simulink library "EmotorLib"  (R2024b)
settings: Solver=VariableStepAuto  StartTime=0.0  StopTime=10.0  RelTol=1e-3
undefined symbols (not defined in the file or in its folder): electricDrive
libraries: fl_lib x56, nesl_utility x11, ee_lib x2
settings Model: Creator=jjha  LastModifiedBy=jjha
settings OptimizationCC: ReuseModelBlockBuffer=off
settings RTWCC: GPUComputeCapability=3.5

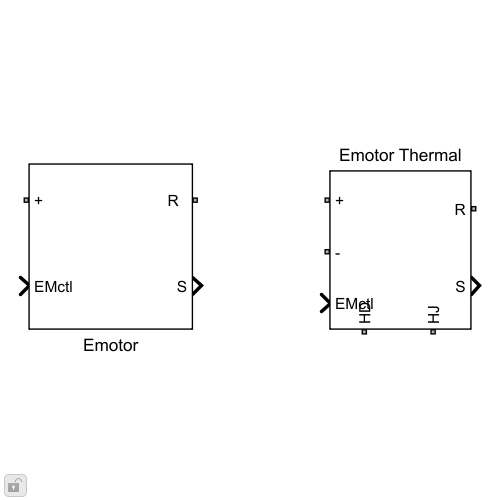
[thumbnail: Simulink's stored preview of the top-level diagram]
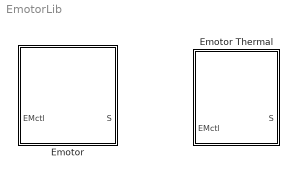
== system EmotorLib ==
  Emotor : Subsystem  mask{max_torque=220, max_power=50000, Tctc=0.002, spMat=[500,10000], tqMat=[10,200], lossMat=[0 0;0 0]}
      mask prompts: max_torque "Max Torque"; max_power "Max Powe"; Tctc "Torque Control Time Constant"; spMat "Speed Vector (rpm)"; tqMat "TorqueVector (Nm)"; lossMat "Losses (W)"
      settings: PortSchema="{\"entries\":[{\"content\":{\"sides\":[{\"content\":{\"connectorIds\":[\"LConn1\",\"In1\"]},\"type\":\"ConnectorPlacement.EquallySpacedRectSide\",\"uuid\":\"4c01f4e7-db0d-4a8e-9bf8-0007797f2983\"},{\"content\":{\"connectorIds\":[\"RConn1\",\"Out1\"],\"side\":\"RIGHT\"},\"type\":\"ConnectorPlacement.EquallySpacedRectSide\",\"uuid\":\"016ff73d-d921-4c23-b0f0-ceb092773eb0\"},{\"content\":{\"connectorIds\":[],\"side\":\"TOP\"},\"type\":\"ConnectorPlacement.EquallySpacedRectSide\",\"uuid\":\"4629c7d5-cdf8-4573-9adc-69c84e237e94\"}]},\"type\":\"ConnectorPlacement.EquallySpacedConnector\",\"uuid\":\"4efbbf6b-ce98-44e7-ad85-9bcf934dac12\"}],\"packageUris\":[\"http://schema.mathworks.com/mf0/Connector/R2020b\"],\"version\":\"1.0\"}"
      mask DialogControl ElecTorque Prompt: Electrical Torque Parameters
      mask DialogControl ElecLosses Prompt: Electrical Losses Parameter
  Emotor Thermal : Subsystem  mask{InitTemp=298.15, IronSpHeat=447, CopperSpHeat=385, IronThConductivity=50, GrossToothMass=0.4836, WindingMass=0.4464, max_torque=220, max_power=50000, Tctc=0.002, spMat=[500,10000], tqMat=[10,200], lossMat=[0 0;0 0], StatorBackIronMass=1.997, StatorRootDia=0.1521, stator_od=0.19812, StatorWindingOhArea=0.0538, Bridgemass=0.0698, rotor_od=.12997, rotorStackLength=0.1516, RotorBackIronMass=16.3802, RotorAreaER=0.0265, RotorAreaCyl=0.0619}
      mask prompts: InitTemp "Initial Temperature(K)"; IronSpHeat "Specific Heat Iron(J/(K*kg))"; CopperSpHeat "Specific Heat Copper(J/(K*kg))"; IronThConductivity "Thermal Conductivity Iron(W/(K*m))"; GrossToothMass "Stator Teeth Mass(kg)"; WindingMass "Stator Winding Mass(kg)"; max_torque "Max Torque"; max_power "Max Power"; Tctc "Torque Control Time Constant"; spMat "Speed Vector (rpm)"; tqMat "TorqueVector (Nm)"; lossMat "Losses (W)"; StatorBackIronMass "Stator Back Iron Mass(kg)"; StatorRootDia "Stator Inner Diameter (m)"; stator_od "Stator Outer Diameter(m)"; StatorWindingOhArea "Stator Winding Area(m^2)"; Bridgemass "Magnet Mass(kg)"; rotor_od "Rotor Outer Diameter(m)"; rotorStackLength "Stack Length(m)"; RotorBackIronMass "Rotor Iron Mass(kg)"; RotorAreaER "Rotor Area ER(m^2)"; RotorAreaCyl "Rotor Cylinder Area(m^2)"
      settings: PortSchema="{\"entries\":[{\"content\":{\"sides\":[{\"content\":{\"connectorIds\":[\"LConn1\",\"LConn2\",\"In1\"]},\"type\":\"ConnectorPlacement.EquallySpacedRectSide\",\"uuid\":\"10df522d-563d-4b08-8533-b994fdc6485c\"},{\"content\":{\"connectorIds\":[\"RConn1\",\"Out1\"],\"side\":\"RIGHT\"},\"type\":\"ConnectorPlacement.EquallySpacedRectSide\",\"uuid\":\"49c7f672-865f-471b-9e0c-89a8670e12b9\"},{\"content\":{\"connectorIds\":[],\"side\":\"TOP\"},\"type\":\"ConnectorPlacement.EquallySpacedRectSide\",\"uuid\":\"483d1bb0-f2a2-4e3e-b03d-59043e33c561\"},{\"content\":{\"connectorIds\":[\"RConn2\",\"RConn3\"],\"side\":\"BOTTOM\"},\"type\":\"ConnectorPlacement.EquallySpacedRectSide\",\"uuid\":\"9824884f-8ef8-4acd-9b94-f9f251c18df1\"}]},\"type\":\"ConnectorPlacement.EquallySpacedConnector\",\"uuid\":\"fbb57d51-9a3c-403f-b1bb-2fd61ef310af\"}],\"packageUris\":[\"http://schema.mathworks.com/mf0/Connector/R2020b\"],\"version\":\"1.0\"}"
      mask DialogControl Container5 Prompt: Electrical Parameters
      mask DialogControl ElecTorque Prompt: Electrical Torque Parameters
      mask DialogControl ElecLosses Prompt: Electrical Losses Parameter
      mask DialogControl Container6 Prompt: Thermal Parameters
      mask DialogControl Container8 Prompt: Rotor
      mask DialogControl Container7 Prompt: Stator

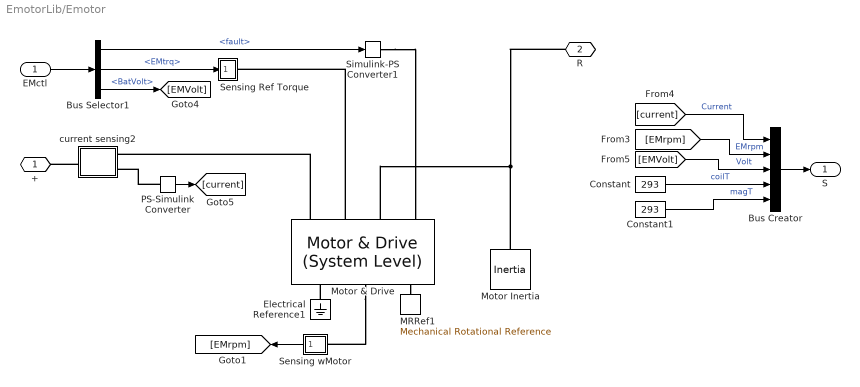
== system EmotorLib/Emotor ==
  EMctl : Inport
  Bus Creator : BusCreator  Inputs=5
  Bus Selector1 : BusSelector  OutputSignals=fault,EMtrq,BatVolt
  Constant : Constant  Value=293
  Constant1 : Constant  Value=293
  Electrical Reference1 : fl_lib/Electrical/Electrical Elements/Electrical Reference
  MRRef1 : fl_lib/Mechanical/Rotational Elements/Mechanical Rotational Reference
  Motor & Drive : ee_lib/Electromechanical/Motor & Drive (System Level)  torque_speed_param=2  overtorque_param=ee.enum.electromech.overtorque.no  T_t=[max_torque max_torque max_torque 0] N*m  T_t_intermittent=[.36, .32, .28, 0] N*m  T_t_2D=[.09, .09, .09; .08, .08, .08; .07, .07, .07; 0, 0, 0] N*m  T_t_intermittent_2D=[.36, .36, .36; .32, .32, .32; .28, .28, .28; 0, 0, 0] N*m  w_t=[ 0 3.75e+3 7.5e+3 8e+3 ] rpm  vdc_t=[6, 12, 24] V  torque_max=max_torque N*m  power_max=max_power W  torque_max_intermittent=0.4 N*m  power_max_intermittent=120 W  time_overtorque=30 s  time_recover=60 s  Tc=Tctc s  EnableSwitch=simscape.enum.onoff.on  losses_param=2  eff=96  w_eff=1500 rpm  T_eff=50 N*m  Piron=200 W  Pbase=0 W  w_eff_vec=spMat rpm  T_eff_vec=tqMat N*m  v_eff_vec=[100, 250, 400] V  losses_mat=lossMat W  efficiency_mat=[95 95 95 95; 95 95 95 95; 95 95 95 95; 95 95 95 95; 95 95 95 95]  losses_mat_3D=ones(5, 4, 3) W  efficiency_mat_3D=95 * ones(5, 4, 3)  Res=0 Ohm  J=0 kg*m^2  lam=1e-5 N*m/(rad/s)  speed0=0 rpm  fault_condition=1  fault_threshold=0.5  faulted_specify=off  faulted_priority=None  faulted=0  faulted_nominal_specify=off  faulted_nominal_value=1  faulted_nominal_unit=1  isSwitchedOff_specify=off  isSwitchedOff_priority=None  isSwitchedOff=0  isSwitchedOff_nominal_specify=off  isSwitchedOff_nominal_value=1  isSwitchedOff_nominal_unit=1  torqueLimitContinuous_specify=off  torqueLimitContinuous_priority=None  torqueLimitContinuous=0 N*m  torqueLimitContinuous_nominal_specify=off  torqueLimitContinuous_nominal_value=1  torqueLimitContinuous_nominal_unit=N*m  alpha=3.93e-3 1/K  Tmeas=25 degC  Tmeas2=125 degC  losses_mat_T2=[1.49, 1.74, 2.49, 3.74; .42, .67, 1.42, 2.67; .06, .31, 1.06, 2.31; .42, .67, 1.42, 2.67; 1.49, 1.74, 2.49, 3.74] W  efficiency_mat_T2=[95, 95, 95, 95; 95, 95, 95, 95; 95, 95, 95, 95; 95, 95, 95, 95; 95, 95, 95, 95]  losses_mat_3D_T2=ones(5, 4, 3) W  efficiency_mat_3D_T2=95 * ones(5, 4, 3)  thermal_mass=100 J/K  initial_temperature=25 degC
      settings: InternalSimscapePortConfiguration="{\"Bottom\":[],\"Left\":[{\"id\":\"Vp\",\"label\":\"+\",\"type\":\"foundation.electrical.electrical\"},{\"id\":\"Tr\",\"label\":\"Tr\",\"type\":\"input\"},{\"id\":\"R\",\"label\":\"R\",\"type\":\"foundation.mechanical.rotational.rotational\"},{\"id\":\"F\",\"label\":\"SW\",\"type\":\"input\"}],\"Right\":[{\"id\":\"Vm\",\"label\":\"-\",\"type\":\"foundation.electrical.electrical\"},{\"id\":\"Omega\",\"label\":\"w\",\"type\":\"output\"},{\"id\":\"C\",\"label\":\"C\",\"type\":\"foundation.mechanical.rotational.rotational\"}],\"Top\":[]}"
  Motor Inertia : fl_lib/Mechanical/Rotational Elements/Inertia  inertia=0.02 kg*m^2  num_ports=foundation.enum.numPorts2.one  w_specify=on  w_priority=High  w=0 rpm  w_nominal_specify=off  w_nominal_value=1  w_nominal_unit=rad/s  t_specify=off  t_priority=High  t=0 N*m  t_nominal_specify=off  t_nominal_value=1  t_nominal_unit=N*m
  PS-Simulink Converter : nesl_utility/PS-Simulink Converter  PhysicalDomain=network_engine_domain  SubClassName=ps_output  LeftPortType=input  RightPortType=output  PseudoPeriodic=off  Frequencies=[]  VectorFormat=inherit  Unit=inherit  AffineConversion=off
  Sensing Ref Torque : Subsystem
  Sensing wMotor : Subsystem
      mask Display: disp('w');
  Simulink-PS Converter1 : nesl_utility/Simulink-PS Converter  PhysicalDomain=network_engine_domain  SubClassName=ps_input  LeftPortType=input  RightPortType=output  PseudoPeriodic=off  Frequencies=[]  NoiseDistribution=none  NoiseParameters=[]  Unit=1  AffineConversion=off  FilteringAndDerivatives=provide  SimscapeFilterOrder=1  InputFilterTimeConstant=0.001  UdotUserProvided=0
  current sensing2 : Subsystem
  + : PMIOPort  Side=Left
  "R  " : PMIOPort  Port=2  Side=Right
  S : Outport
  wires:
  PS-Simulink Converter/1 -> [current]
  Bus Selector1/2 -> Sensing Ref Torque/1(" ")  "<EMtrq>"
  EMctl/1 -> Bus Selector1/1
  Bus Selector1/3 -> [EMVolt]  "<BatVolt>"
  Bus Selector1/1 -> Simulink-PS Converter1/1  "<fault>"
  [EMVolt] -> Bus Creator/3  "Volt"
  Constant/1 -> Bus Creator/4  "coilT"
  [EMrpm] -> Bus Creator/2  "EMrpm"
  Bus Creator/1 -> S/1
  [current] -> Bus Creator/1  "Current"
  Constant1/1 -> Bus Creator/5  "magT"
  Sensing wMotor/1(SL) -> [EMrpm]
  connections:
  PS-Simulink Converter/LConn1 -- current sensing2/RConn2
  Simulink-PS Converter1/RConn1 -- Motor & Drive/LConn4
  Electrical Reference1/LConn1 -- Motor & Drive/RConn1
  Motor & Drive/RConn2 -- Sensing wMotor/LConn1
  Motor & Drive/LConn2 -- Sensing Ref Torque/RConn1
  current sensing2/LConn1 -- +/RConn1
  Motor & Drive/LConn3 -- "R  "/RConn1 -- Motor Inertia/LConn1
  Motor & Drive/LConn1 -- current sensing2/RConn1
  Motor & Drive/RConn3 -- MRRef1/LConn1

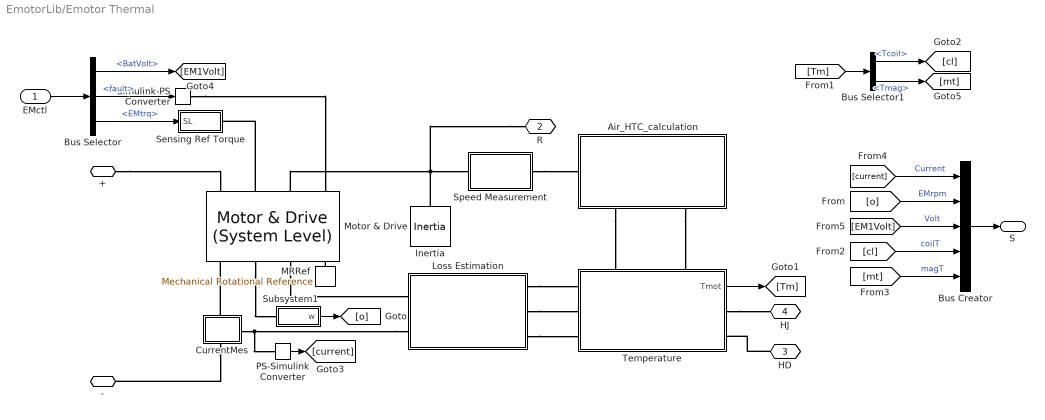
== system EmotorLib/Emotor Thermal ==
  EMctl : Inport
  Air_HTC_calculation : Subsystem
      settings: PortSchema="{\"entries\":[{\"content\":{\"sides\":[{\"content\":{\"connectorIds\":[\"LConn1\"]},\"type\":\"ConnectorPlacement.EquallySpacedRectSide\",\"uuid\":\"c3fc49c2-0151-484f-b0d8-f4e4a060bcaf\"},{\"content\":{\"connectorIds\":[],\"side\":\"RIGHT\"},\"type\":\"ConnectorPlacement.EquallySpacedRectSide\",\"uuid\":\"c73251fe-fcad-4c5f-9d27-fb7ac98c9b31\"},{\"content\":{\"connectorIds\":[],\"side\":\"TOP\"},\"type\":\"ConnectorPlacement.EquallySpacedRectSide\",\"uuid\":\"06ea8515-c1b4-4445-9ea2-9a6fe3b8d822\"},{\"content\":{\"connectorIds\":[\"RConn1\",\"RConn2\"],\"side\":\"BOTTOM\"},\"type\":\"ConnectorPlacement.EquallySpacedRectSide\",\"uuid\":\"0d77474d-64a7-49ab-b2b5-eb3962b26dfa\"}]},\"type\":\"ConnectorPlacement.EquallySpacedConnector\",\"uuid\":\"651eda7a-2416-4496-9b8b-1b2d725cf6dd\"}],\"packageUris\":[\"http://schema.mathworks.com/mf0/Connector/R2020b\"],\"version\":\"1.0\"}"
  Bus Creator : BusCreator  Inputs=5
  Bus Selector : BusSelector  OutputSignals=BatVolt,fault,EMtrq
  Bus Selector1 : BusSelector  OutputSignals=Tcoil,Tmag
  CurrentMes : Subsystem
      settings: PortSchema="{\"entries\":[{\"content\":{\"sides\":[{\"content\":{\"connectorIds\":[\"LConn1\"]},\"type\":\"ConnectorPlacement.EquallySpacedRectSide\",\"uuid\":\"aec73178-3b68-40df-935a-7f5359bce9cd\"},{\"content\":{\"connectorIds\":[],\"side\":\"RIGHT\"},\"type\":\"ConnectorPlacement.EquallySpacedRectSide\",\"uuid\":\"aa898e43-8a60-4280-99e9-69a0b0908b52\"},{\"content\":{\"connectorIds\":[\"LConn2\"],\"side\":\"TOP\"},\"type\":\"ConnectorPlacement.EquallySpacedRectSide\",\"uuid\":\"450895ec-a170-4755-8b37-3fd418fe4f7c\"},{\"content\":{\"connectorIds\":[\"RConn1\"],\"side\":\"BOTTOM\"},\"type\":\"ConnectorPlacement.EquallySpacedRectSide\",\"uuid\":\"50e67d36-6ee8-4450-bc7a-5decbfd7b4fc\"}]},\"type\":\"ConnectorPlacement.EquallySpacedConnector\",\"uuid\":\"d52bc816-e8fd-442f-9361-ac497bbc1898\"}],\"packageUris\":[\"http://schema.mathworks.com/mf0/Connector/R2020b\"],\"version\":\"1.0\"}"
  Inertia : fl_lib/Mechanical/Rotational Elements/Inertia  inertia=0.02 kg*m^2  num_ports=foundation.enum.numPorts2.one  w_specify=on  w_priority=High  w=0 rad/s  w_nominal_specify=off  w_nominal_value=1  w_nominal_unit=rad/s  t_specify=off  t_priority=None  t=0 N*m  t_nominal_specify=off  t_nominal_value=1  t_nominal_unit=N*m
  Loss Estimation : Subsystem
  MRRef : fl_lib/Mechanical/Rotational Elements/Mechanical Rotational Reference
  Motor & Drive : ee_lib/Electromechanical/Motor & Drive (System Level)  torque_speed_param=2  overtorque_param=ee.enum.electromech.overtorque.no  T_t=[max_torque max_torque max_torque 0] N*m  T_t_intermittent=[.36, .32, .28, 0] N*m  T_t_2D=[.09, .09, .09; .08, .08, .08; .07, .07, .07; 0, 0, 0] N*m  T_t_intermittent_2D=[.36, .36, .36; .32, .32, .32; .28, .28, .28; 0, 0, 0] N*m  w_t=[ 0 3.75e+3 7.5e+3 8e+3 ] rpm  vdc_t=[6, 12, 24] V  torque_max=electricDrive.max_torque N*m  power_max=electricDrive.max_power W  torque_max_intermittent=0.4 N*m  power_max_intermittent=120 W  time_overtorque=30 s  time_recover=60 s  Tc=electricDrive.Tctc s  EnableSwitch=simscape.enum.onoff.on  losses_param=2  eff=96  w_eff=1500 rpm  T_eff=50 N*m  Piron=200 W  Pbase=0 W  w_eff_vec=electricDrive.motor_loss_map.spMat rpm  T_eff_vec="electricDrive.motor_loss_map.tqMat      N*m"  v_eff_vec=[100, 250, 400] V  losses_mat=electricDrive.motor_loss_map.lossMat W  efficiency_mat=[95 95 95 95; 95 95 95 95; 95 95 95 95; 95 95 95 95; 95 95 95 95]  losses_mat_3D=ones(5, 4, 3) W  efficiency_mat_3D=95 * ones(5, 4, 3)  Res=0 Ohm  J=0 kg*m^2  lam=1e-5 N*m/(rad/s)  speed0=0 rpm  fault_condition=1  fault_threshold=0.5  faulted_specify=off  faulted_priority=None  faulted=0  faulted_nominal_specify=off  faulted_nominal_value=1  faulted_nominal_unit=1  isSwitchedOff_specify=off  isSwitchedOff_priority=None  isSwitchedOff=0  isSwitchedOff_nominal_specify=off  isSwitchedOff_nominal_value=1  isSwitchedOff_nominal_unit=1  torqueLimitContinuous_specify=off  torqueLimitContinuous_priority=None  torqueLimitContinuous=0 N*m  torqueLimitContinuous_nominal_specify=off  torqueLimitContinuous_nominal_value=1  torqueLimitContinuous_nominal_unit=N*m  alpha=0.00393 1/K  Tmeas=298.15 degC  Tmeas2=398.15 degC  losses_mat_T2=electricDrive.motor_loss_map.lossMat W  efficiency_mat_T2=[95 95 95 95; 95 95 95 95; 95 95 95 95; 95 95 95 95; 95 95 95 95]  losses_mat_3D_T2=ones(5, 4, 3) W  efficiency_mat_3D_T2=95 * ones(5, 4, 3)  thermal_mass=15000 J/K  initial_temperature=298.15 K
      settings: InternalSimscapePortConfiguration="{\"Bottom\":[],\"Left\":[{\"id\":\"Vp\",\"label\":\"+\",\"type\":\"foundation.electrical.electrical\"},{\"id\":\"Tr\",\"label\":\"Tr\",\"type\":\"input\"},{\"id\":\"R\",\"label\":\"R\",\"type\":\"foundation.mechanical.rotational.rotational\"},{\"id\":\"F\",\"label\":\"SW\",\"type\":\"input\"}],\"Right\":[{\"id\":\"Vm\",\"label\":\"-\",\"type\":\"foundation.electrical.electrical\"},{\"id\":\"Omega\",\"label\":\"w\",\"type\":\"output\"},{\"id\":\"H\",\"label\":\"H\",\"type\":\"foundation.thermal.thermal\"},{\"id\":\"C\",\"label\":\"C\",\"type\":\"foundation.mechanical.rotational.rotational\"}],\"Top\":[]}"
  PS-Simulink Converter : nesl_utility/PS-Simulink Converter  PhysicalDomain=network_engine_domain  SubClassName=ps_output  LeftPortType=input  RightPortType=output  PseudoPeriodic=off  Frequencies=[]  VectorFormat=inherit  Unit=inherit  AffineConversion=off
  Sensing Ref Torque : Subsystem
      mask Display: disp('trqRef')
  Simulink-PS Converter : nesl_utility/Simulink-PS Converter  PhysicalDomain=network_engine_domain  SubClassName=ps_input  LeftPortType=input  RightPortType=output  PseudoPeriodic=off  Frequencies=[]  NoiseDistribution=none  NoiseParameters=[]  Unit=1  AffineConversion=off  FilteringAndDerivatives=provide  SimscapeFilterOrder=1  InputFilterTimeConstant=0.001  UdotUserProvided=0
  Speed Measurement : Subsystem
  Subsystem1 : Subsystem
      settings: PortSchema="{\"entries\":[{\"content\":{\"sides\":[{\"content\":{},\"type\":\"ConnectorPlacement.EquallySpacedRectSide\",\"uuid\":\"73dca2aa-f399-4eeb-9d48-20c826d2ded4\"},{\"content\":{\"side\":\"RIGHT\"},\"type\":\"ConnectorPlacement.EquallySpacedRectSide\",\"uuid\":\"ff117f44-2f45-4c10-9502-0d11ada2d007\"},{\"content\":{\"connectorIds\":[\"LConn1\"],\"side\":\"TOP\"},\"type\":\"ConnectorPlacement.EquallySpacedRectSide\",\"uuid\":\"808df778-70a2-4117-a4b0-06aebafa20a3\"},{\"content\":{\"connectorIds\":[\"Out1\"],\"side\":\"BOTTOM\"},\"type\":\"ConnectorPlacement.EquallySpacedRectSide\",\"uuid\":\"ea26dad2-5611-48d3-b3ad-420e5e152393\"}]},\"type\":\"ConnectorPlacement.EquallySpacedConnector\",\"uuid\":\"b8b92b14-f871-4df7-89f6-65702e38d2f7\"}],\"packageUris\":[\"http://schema.mathworks.com/mf0/Connector/R2020b\"],\"version\":\"1.0\"}"
  Temperature : Subsystem
      settings: PortSchema="{\"entries\":[{\"content\":{\"sides\":[{\"content\":{\"connectorIds\":[\"LConn1\",\"LConn2\",\"LConn3\"]},\"type\":\"ConnectorPlacement.EquallySpacedRectSide\",\"uuid\":\"fee72484-960d-4cd4-9296-e38678962aa1\"},{\"content\":{\"connectorIds\":[\"Out1\",\"RConn1\",\"RConn2\"],\"side\":\"RIGHT\"},\"type\":\"ConnectorPlacement.EquallySpacedRectSide\",\"uuid\":\"5fc115b4-63fd-47d3-871d-1c82ac52ac43\"},{\"content\":{\"connectorIds\":[\"LConn4\",\"LConn5\"],\"side\":\"TOP\"},\"type\":\"ConnectorPlacement.EquallySpacedRectSide\",\"uuid\":\"406f719a-f995-4122-9f35-24e8332a2e84\"},{\"content\":{\"connectorIds\":[],\"side\":\"BOTTOM\"},\"type\":\"ConnectorPlacement.EquallySpacedRectSide\",\"uuid\":\"14dc85e6-8157-4b38-8651-862ce77721cd\"}]},\"type\":\"ConnectorPlacement.EquallySpacedConnector\",\"uuid\":\"1dcc2b5d-90fd-40de-873d-99118eb86bdd\"}],\"packageUris\":[\"http://schema.mathworks.com/mf0/Connector/R2020b\"],\"version\":\"1.0\"}"
  + : PMIOPort  Side=Left
  R : PMIOPort  Port=2  Side=Right
  HD : PMIOPort  Port=3  Side=Right
  HJ : PMIOPort  Port=4  Side=Right
  - : PMIOPort  Port=5  Side=Left
  S : Outport
  wires:
  [EM1Volt] -> Bus Creator/3  "Volt"
  Bus Selector/3 -> Sensing Ref Torque/1(SL)  "<EMtrq>"
  [Tm] -> Bus Selector1/1
  Subsystem1/1(w) -> [o]
  Bus Selector/2 -> Simulink-PS Converter/1  "<fault>"
  PS-Simulink Converter/1 -> [current]
  Temperature/1(Tmot) -> [Tm]
  Bus Creator/1 -> S/1
  Bus Selector/1 -> [EM1Volt]  "<BatVolt>"
  [current] -> Bus Creator/1  "Current"
  [mt] -> Bus Creator/5  "magT"
  [cl] -> Bus Creator/4  "coilT"
  EMctl/1 -> Bus Selector/1
  Bus Selector1/1 -> [cl]  "<Tcoil>"
  Bus Selector1/2 -> [mt]  "<Tmag>"
  [o] -> Bus Creator/2  "EMrpm"
  connections:
  R/RConn1 -- Inertia/LConn1 -- Speed Measurement/LConn1 -- Motor & Drive/LConn3
  Loss Estimation/LConn2 -- PS-Simulink Converter/LConn1 -- CurrentMes/LConn1
  Air_HTC_calculation/RConn2 -- Temperature/LConn5
  Loss Estimation/RConn3 -- Temperature/LConn3
  +/RConn1 -- Motor & Drive/LConn1
  Temperature/RConn1 -- HJ/RConn1
  CurrentMes/LConn2 -- Motor & Drive/RConn1
  MRRef/LConn1 -- Motor & Drive/RConn4
  Loss Estimation/RConn2 -- Temperature/LConn2
  Loss Estimation/RConn1 -- Temperature/LConn1
  Speed Measurement/RConn1 -- Air_HTC_calculation/LConn1
  Motor & Drive/RConn2 -- Subsystem1/LConn1
  Motor & Drive/LConn2 -- Sensing Ref Torque/RConn1
  Air_HTC_calculation/RConn1 -- Temperature/LConn4
  CurrentMes/RConn1 -- -/RConn1
  HD/RConn1 -- Temperature/RConn2
  Simulink-PS Converter/RConn1 -- Motor & Drive/LConn4
  Motor & Drive/RConn3 -- Loss Estimation/LConn1

== system EmotorLib/Emotor/Sensing Ref Torque ==
  " " : Inport
  Simulink-PS G1 : nesl_utility/Simulink-PS Converter  PhysicalDomain=network_engine_domain  SubClassName=ps_input  LeftPortType=input  RightPortType=output  PseudoPeriodic=off  Frequencies=[]  NoiseDistribution=none  NoiseParameters=[]  Unit=N*m  AffineConversion=off  FilteringAndDerivatives=zero  SimscapeFilterOrder=1  InputFilterTimeConstant=1e-6  UdotUserProvided=1
  "  " : PMIOPort  Side=Right
  wires:
  " "/1 -> Simulink-PS G1/1
  connections:
  Simulink-PS G1/RConn1 -- "  "/RConn1

== system EmotorLib/Emotor/Sensing wMotor ==
  PS-Simulink Converter : nesl_utility/PS-Simulink Converter  PhysicalDomain=network_engine_domain  SubClassName=ps_output  LeftPortType=input  RightPortType=output  PseudoPeriodic=off  Frequencies=[]  VectorFormat=1-D array  Unit=rpm  AffineConversion=off
  PS : PMIOPort  Side=Left
  SL : Outport  VectorParamsAs1DForOutWhenUnconnected=off
  wires:
  PS-Simulink Converter/1 -> SL/1
  connections:
  PS/RConn1 -- PS-Simulink Converter/LConn1

== system EmotorLib/Emotor/current sensing2 ==
  Current Sensor : fl_lib/Electrical/Electrical Sensors/Current Sensor
  " " : PMIOPort  Side=Left
  "  " : PMIOPort  Port=2  Side=Right
  "  I" : PMIOPort  Port=3  Side=Right
  connections:
  Current Sensor/RConn1 -- "  I"/RConn1
  Current Sensor/LConn1 -- " "/RConn1
  Current Sensor/RConn2 -- "  "/RConn1

== system EmotorLib/Emotor Thermal/Air_HTC_calculation ==
  Rotor side  HTC : Subsystem
  Rotor_Taylor_Couette  HTC : Subsystem
  w : PMIOPort  Side=Left
  HTC_TC : PMIOPort  Port=2  Side=Right
  HTC : PMIOPort  Port=3  Side=Right
  connections:
  Rotor side  HTC/LConn1 -- w/RConn1 -- Rotor_Taylor_Couette  HTC/LConn1
  HTC/RConn1 -- Rotor side  HTC/RConn1
  Rotor_Taylor_Couette  HTC/RConn1 -- HTC_TC/RConn1

== system EmotorLib/Emotor Thermal/CurrentMes ==
  Current Sensor : fl_lib/Electrical/Electrical Sensors/Current Sensor
  I : PMIOPort  Side=Left
  + : PMIOPort  Port=2  Side=Left
  - : PMIOPort  Port=3  Side=Right
  connections:
  -/RConn1 -- Current Sensor/RConn2
  Current Sensor/RConn1 -- I/RConn1
  Current Sensor/LConn1 -- +/RConn1

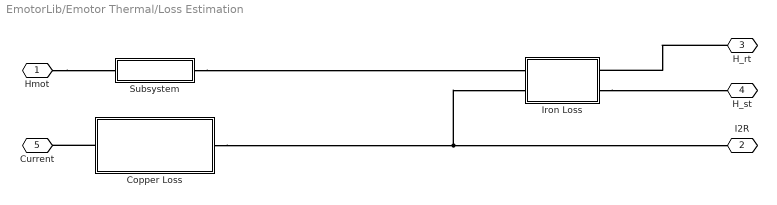
== system EmotorLib/Emotor Thermal/Loss Estimation ==
  "Copper Loss " : Subsystem
  Iron Loss : Subsystem
  Subsystem : Subsystem
  Hmot : PMIOPort  Side=Left
  I2R : PMIOPort  Port=2  Side=Right
  H_rt : PMIOPort  Port=3  Side=Right
  H_st : PMIOPort  Port=4  Side=Right
  Current : PMIOPort  Port=5  Side=Left
  connections:
  H_rt/RConn1 -- Iron Loss/RConn1
  Iron Loss/RConn2 -- H_st/RConn1
  Hmot/RConn1 -- Subsystem/LConn1
  "Copper Loss "/LConn1 -- Current/RConn1
  "Copper Loss "/RConn1 -- Iron Loss/LConn2 -- I2R/RConn1
  Subsystem/RConn1 -- Iron Loss/LConn1

== system EmotorLib/Emotor Thermal/Sensing Ref Torque ==
  SL : Inport
  Simulink-PS G1 : nesl_utility/Simulink-PS Converter  PhysicalDomain=network_engine_domain  SubClassName=ps_input  LeftPortType=input  RightPortType=output  PseudoPeriodic=off  Frequencies=[]  NoiseDistribution=none  NoiseParameters=[]  Unit=N*m  AffineConversion=off  FilteringAndDerivatives=zero  SimscapeFilterOrder=1  InputFilterTimeConstant=1e-6  UdotUserProvided=1
  PS : PMIOPort  Side=Right
  wires:
  SL/1 -> Simulink-PS G1/1
  connections:
  Simulink-PS G1/RConn1 -- PS/RConn1

== system EmotorLib/Emotor Thermal/Speed Measurement ==
  Ideal Rotational Motion Sensor : fl_lib/Mechanical/Mechanical Sensors/Ideal Rotational Motion Sensor  reference=foundation.enum.MeasurementReference.difference  acceleration_port=false  velocity_port=true  position_port=false  wrap_angle=false  offset=0 rad
      settings: InternalSimscapePortConfiguration="{\"Bottom\":[],\"Left\":[{\"id\":\"R\",\"label\":\"R\",\"type\":\"foundation.mechanical.rotational.rotational\"}],\"Right\":[{\"id\":\"C\",\"label\":\"C\",\"type\":\"foundation.mechanical.rotational.rotational\"},{\"id\":\"W\",\"label\":\"W\",\"type\":\"output\"}],\"Top\":[]}"
  MRRef1 : fl_lib/Mechanical/Rotational Elements/Mechanical Rotational Reference
  spd : PMIOPort  Side=Right
  mot : PMIOPort  Port=2  Side=Left
  connections:
  MRRef1/LConn1 -- Ideal Rotational Motion Sensor/RConn1
  mot/RConn1 -- Ideal Rotational Motion Sensor/LConn1
  spd/RConn1 -- Ideal Rotational Motion Sensor/RConn2

== system EmotorLib/Emotor Thermal/Subsystem1 ==
  Sensing wMotor : Subsystem
      mask Display: disp('w');
  PS : PMIOPort  Side=Left
  w : Outport  VectorParamsAs1DForOutWhenUnconnected=off
  wires:
  Sensing wMotor/1(SL) -> w/1
  connections:
  PS/RConn1 -- Sensing wMotor/LConn1

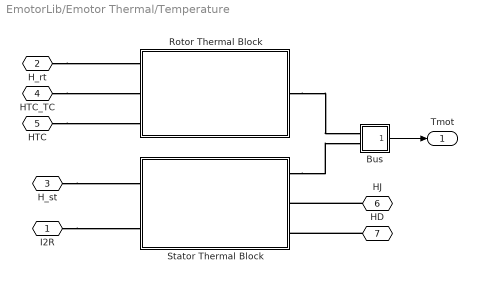
== system EmotorLib/Emotor Thermal/Temperature ==
  Bus : Subsystem
  Rotor Thermal Block : Subsystem
  Stator Thermal Block : Subsystem
  I2R : PMIOPort  Side=Left
  H_rt : PMIOPort  Port=2  Side=Left
  H_st : PMIOPort  Port=3  Side=Left
  HTC_TC : PMIOPort  Port=4  Side=Left
  HTC : PMIOPort  Port=5  Side=Left
  HJ : PMIOPort  Port=6  Side=Right
  HD : PMIOPort  Port=7  Side=Right
  Tmot : Outport
  wires:
  Bus/1("   ") -> Tmot/1
  connections:
  HJ/RConn1 -- Stator Thermal Block/LConn2
  H_rt/RConn1 -- Rotor Thermal Block/RConn1
  H_st/RConn1 -- Stator Thermal Block/RConn1
  I2R/RConn1 -- Stator Thermal Block/RConn2
  HTC_TC/RConn1 -- Rotor Thermal Block/RConn2
  HTC/RConn1 -- Rotor Thermal Block/RConn3
  Rotor Thermal Block/LConn1 -- Bus/LConn1
  Stator Thermal Block/LConn1 -- Bus/LConn2
  HD/RConn1 -- Stator Thermal Block/LConn3

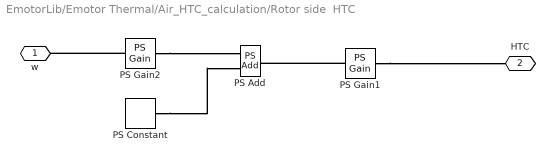
== system EmotorLib/Emotor Thermal/Air_HTC_calculation/Rotor side  HTC ==
  PS Add : fl_lib/Physical Signals/Functions/PS Add
  PS Constant : fl_lib/Physical Signals/Sources/PS Constant  constant=8.1387 rad/s
  PS Gain1 : fl_lib/Physical Signals/Functions/PS Gain  gain=2.217 W*s/(m^2*K*rad)
  PS Gain2 : fl_lib/Physical Signals/Functions/PS Gain  gain=0.0265
  w : PMIOPort  Side=Left
  HTC : PMIOPort  Port=2  Side=Right
  connections:
  PS Gain2/LConn1 -- w/RConn1
  PS Gain1/RConn1 -- HTC/RConn1
  PS Gain1/LConn1 -- PS Add/RConn1
  PS Gain2/RConn1 -- PS Add/LConn1
  PS Constant/RConn1 -- PS Add/LConn2

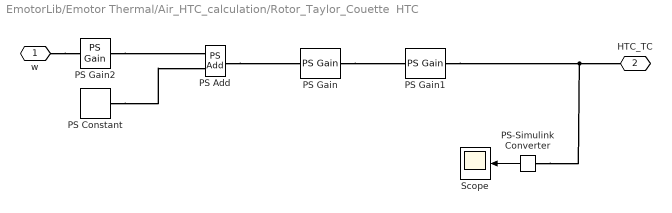
== system EmotorLib/Emotor Thermal/Air_HTC_calculation/Rotor_Taylor_Couette  HTC ==
  PS Add : fl_lib/Physical Signals/Functions/PS Add
  PS Constant : fl_lib/Physical Signals/Sources/PS Constant  constant=8.1387 rad/s
  PS Gain : fl_lib/Physical Signals/Functions/PS Gain  gain=2.667e-6 s/rad
  PS Gain1 : fl_lib/Physical Signals/Functions/PS Gain  gain=1 W/(m^2*K)
  PS Gain2 : fl_lib/Physical Signals/Functions/PS Gain  gain=0.0265
  PS-Simulink Converter : nesl_utility/PS-Simulink Converter  PhysicalDomain=network_engine_domain  SubClassName=ps_output  LeftPortType=input  RightPortType=output  PseudoPeriodic=off  Frequencies=[]  VectorFormat=inherit  Unit=inherit  AffineConversion=off
  Scope : Scope
  w : PMIOPort  Side=Left
  HTC_TC : PMIOPort  Port=2  Side=Right
  wires:
  PS-Simulink Converter/1 -> Scope/1
  connections:
  PS Gain/RConn1 -- PS Gain1/LConn1
  w/RConn1 -- PS Gain2/LConn1
  PS Gain1/RConn1 -- PS-Simulink Converter/LConn1 -- HTC_TC/RConn1
  PS Gain2/RConn1 -- PS Add/LConn1
  PS Constant/RConn1 -- PS Add/LConn2
  PS Add/RConn1 -- PS Gain/LConn1

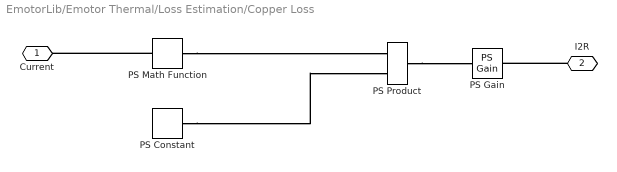
== system EmotorLib/Emotor Thermal/Loss Estimation/Copper Loss  ==
  PS Constant : fl_lib/Physical Signals/Sources/PS Constant  constant=0.0103 Ohm
  PS Gain : fl_lib/Physical Signals/Functions/PS Gain  gain=1
  PS Math Function : fl_lib/Physical Signals/Functions/PS Math Function  fcn_choice=foundation.enum.math_function.square  v=1
  PS Product : fl_lib/Physical Signals/Functions/PS Product
  Current : PMIOPort  Side=Left
  I2R : PMIOPort  Port=2  Side=Right
  connections:
  PS Math Function/LConn1 -- Current/RConn1
  PS Constant/RConn1 -- PS Product/LConn2
  PS Math Function/RConn1 -- PS Product/LConn1
  PS Product/RConn1 -- PS Gain/LConn1
  I2R/RConn1 -- PS Gain/RConn1

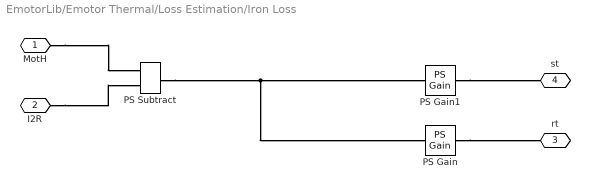
== system EmotorLib/Emotor Thermal/Loss Estimation/Iron Loss ==
  PS Gain : fl_lib/Physical Signals/Functions/PS Gain  gain=electricDrive.MotorThermal.vFractBridge*0.4
  PS Gain1 : fl_lib/Physical Signals/Functions/PS Gain  gain=electricDrive.MotorThermal.vFractTooth*1.1
  PS Subtract : fl_lib/Physical Signals/Functions/PS Subtract
  MotH : PMIOPort  Side=Left
  I2R : PMIOPort  Port=2  Side=Left
  rt : PMIOPort  Port=3  Side=Right
  st : PMIOPort  Port=4  Side=Right
  connections:
  MotH/RConn1 -- PS Subtract/LConn1
  I2R/RConn1 -- PS Subtract/LConn2
  PS Subtract/RConn1 -- PS Gain/LConn1 -- PS Gain1/LConn1
  PS Gain/RConn1 -- rt/RConn1
  PS Gain1/RConn1 -- st/RConn1

== system EmotorLib/Emotor Thermal/Loss Estimation/Subsystem ==
  Heat Flow Rate Sensor : fl_lib/Thermal/Thermal Sensors/Heat Flow Rate Sensor
  Temperature Source : fl_lib/Thermal/Thermal Sources/Temperature Source  temperature=298.15 K
  Hmot : PMIOPort  Side=Left
  MotH : PMIOPort  Port=2  Side=Right
  connections:
  MotH/RConn1 -- Heat Flow Rate Sensor/RConn1
  Hmot/RConn1 -- Heat Flow Rate Sensor/LConn1
  Temperature Source/LConn1 -- Heat Flow Rate Sensor/RConn2

== system EmotorLib/Emotor Thermal/Subsystem1/Sensing wMotor ==
  PS-Simulink Converter : nesl_utility/PS-Simulink Converter  PhysicalDomain=network_engine_domain  SubClassName=ps_output  LeftPortType=input  RightPortType=output  PseudoPeriodic=off  Frequencies=[]  VectorFormat=1-D array  Unit=rpm  AffineConversion=off
  PS : PMIOPort  Side=Left
  SL : Outport  VectorParamsAs1DForOutWhenUnconnected=off
  wires:
  PS-Simulink Converter/1 -> SL/1
  connections:
  PS/RConn1 -- PS-Simulink Converter/LConn1

== system EmotorLib/Emotor Thermal/Temperature/Bus ==
  Bus Creator : BusCreator  Inputs=2
  PS-Simulink Converter : nesl_utility/PS-Simulink Converter  PhysicalDomain=network_engine_domain  SubClassName=ps_output  LeftPortType=input  RightPortType=output  PseudoPeriodic=off  Frequencies=[]  VectorFormat=inherit  Unit=inherit  AffineConversion=off
  PS-Simulink Converter1 : nesl_utility/PS-Simulink Converter  PhysicalDomain=network_engine_domain  SubClassName=ps_output  LeftPortType=input  RightPortType=output  PseudoPeriodic=off  Frequencies=[]  VectorFormat=inherit  Unit=inherit  AffineConversion=off
  " " : PMIOPort  Side=Left
  "  " : PMIOPort  Port=2  Side=Left
  "   " : Outport
  wires:
  PS-Simulink Converter1/1 -> Bus Creator/2  "Tcoil"
  PS-Simulink Converter/1 -> Bus Creator/1  "Tmag"
  Bus Creator/1 -> "   "/1
  connections:
  "  "/RConn1 -- PS-Simulink Converter1/LConn1
  " "/RConn1 -- PS-Simulink Converter/LConn1

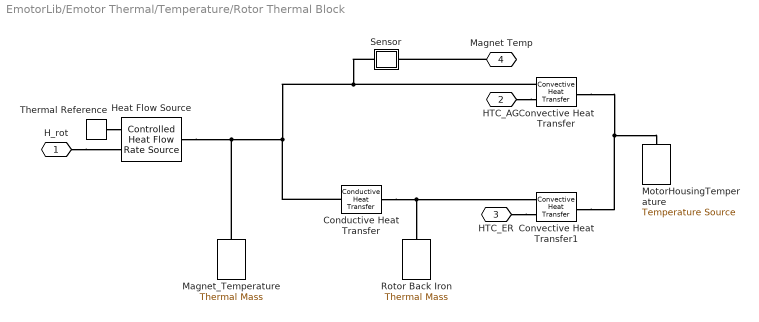
== system EmotorLib/Emotor Thermal/Temperature/Rotor Thermal Block ==
  Conductive Heat Transfer : fl_lib/Thermal/Thermal Elements/Conductive Heat Transfer  thermal_type=foundation.enum.ConstantVariableTabulated.Constant  wall_geometry=foundation.enum.ConductionWallGeometry.Cylindrical  area=1e-4 m^2  thickness=0.1 m  d_in=0.005 m  d_out=rotor_od m  L=rotorStackLength m  th_cond_min=10 W/(K*m)  th_cond=IronThConductivity W/(K*m)  th_cond_TLU=[413, 401, 392, 383, 371, 357, 342] W/(K*m)  temp_TLU=[200, 273, 400, 600, 800, 1000, 1200] K  T_specify=off  T_priority=None  T=0 K  T_nominal_specify=off  T_nominal_value=1  T_nominal_unit=K  Q_specify=off  Q_priority=None  Q=0 W  Q_nominal_specify=off  Q_nominal_value=1  Q_nominal_unit=W
  Convective Heat Transfer : fl_lib/Thermal/Thermal Elements/Convective Heat Transfer  thermal_type=foundation.enum.constant_variable.variable  area=RotorAreaCyl m^2  heat_tr_coeff=10 W/(K*m^2)  min_heat_tr_coeff=1e-3 W/(K*m^2)  T_specify=off  T_priority=None  T=0 K  T_nominal_specify=off  T_nominal_value=1  T_nominal_unit=K  Q_specify=off  Q_priority=None  Q=0 W  Q_nominal_specify=off  Q_nominal_value=1  Q_nominal_unit=W
      settings: InternalSimscapePortConfiguration="{\"Bottom\":[],\"Left\":[{\"id\":\"A\",\"label\":\"A\",\"type\":\"foundation.thermal.thermal\"},{\"id\":\"var_heat_tr_coeff\",\"label\":\"K\",\"type\":\"input\"}],\"Right\":[{\"id\":\"B\",\"label\":\"B\",\"type\":\"foundation.thermal.thermal\"}],\"Top\":[]}"
  Convective Heat Transfer1 : fl_lib/Thermal/Thermal Elements/Convective Heat Transfer  thermal_type=foundation.enum.constant_variable.variable  area=RotorAreaER m^2  heat_tr_coeff=20 W/(K*m^2)  min_heat_tr_coeff=1e-3 W/(K*m^2)  T_specify=off  T_priority=None  T=0 K  T_nominal_specify=off  T_nominal_value=1  T_nominal_unit=K  Q_specify=off  Q_priority=None  Q=0 W  Q_nominal_specify=off  Q_nominal_value=1  Q_nominal_unit=W
      settings: InternalSimscapePortConfiguration="{\"Bottom\":[],\"Left\":[{\"id\":\"A\",\"label\":\"A\",\"type\":\"foundation.thermal.thermal\"},{\"id\":\"var_heat_tr_coeff\",\"label\":\"K\",\"type\":\"input\"}],\"Right\":[{\"id\":\"B\",\"label\":\"B\",\"type\":\"foundation.thermal.thermal\"}],\"Top\":[]}"
  Heat Flow Source : fl_lib/Thermal/Thermal Sources/Controlled Heat Flow Rate Source
  "Magnet_Temperature " : fl_lib/Thermal/Thermal Elements/Thermal Mass  mass_type=foundation.enum.constant_variable.constant  mass=Bridgemass kg  sp_heat=IronSpHeat J/(K*kg)  mass_min=1e-6 kg  num_ports=foundation.enum.numPorts2.one  m_specify=off  m_priority=High  m=1 kg  m_nominal_specify=off  m_nominal_value=1  m_nominal_unit=kg  T_specify=on  T_priority=High  T=InitTemp K  T_nominal_specify=off  T_nominal_value=1  T_nominal_unit=K  Q_specify=off  Q_priority=None  Q=0 W  Q_nominal_specify=off  Q_nominal_value=1  Q_nominal_unit=W
  MotorHousingTemperature : fl_lib/Thermal/Thermal Sources/Temperature Source  temperature=90 degC
  Rotor Back Iron : fl_lib/Thermal/Thermal Elements/Thermal Mass  mass_type=foundation.enum.constant_variable.constant  mass=RotorBackIronMass kg  sp_heat=IronSpHeat J/(K*kg)  mass_min=1e-6 kg  num_ports=foundation.enum.numPorts2.one  m_specify=off  m_priority=High  m=1 kg  m_nominal_specify=off  m_nominal_value=1  m_nominal_unit=kg  T_specify=on  T_priority=High  T=InitTemp K  T_nominal_specify=off  T_nominal_value=1  T_nominal_unit=K  Q_specify=off  Q_priority=None  Q=0 W  Q_nominal_specify=off  Q_nominal_value=1  Q_nominal_unit=W
  Sensor : Subsystem
  Thermal Reference : fl_lib/Thermal/Thermal Elements/Thermal Reference
  H_rot : PMIOPort  Side=Right
  HTC_AG : PMIOPort  Port=2  Side=Right
  HTC_ER : PMIOPort  Port=3  Side=Right
  Magnet Temp : PMIOPort  Port=4  Side=Left
  connections:
  Thermal Reference/LConn1 -- Heat Flow Source/RConn2
  Conductive Heat Transfer/RConn1 -- Convective Heat Transfer1/LConn1 -- Rotor Back Iron/LConn1
  Convective Heat Transfer/RConn1 -- Convective Heat Transfer1/RConn1 -- MotorHousingTemperature/LConn1
  Heat Flow Source/LConn1 -- "Magnet_Temperature "/LConn1 -- Conductive Heat Transfer/LConn1 -- Sensor/LConn1 -- Convective Heat Transfer/LConn1
  HTC_AG/RConn1 -- Convective Heat Transfer/LConn2
  HTC_ER/RConn1 -- Convective Heat Transfer1/LConn2
  H_rot/RConn1 -- Heat Flow Source/RConn1
  Magnet Temp/RConn1 -- Sensor/RConn1

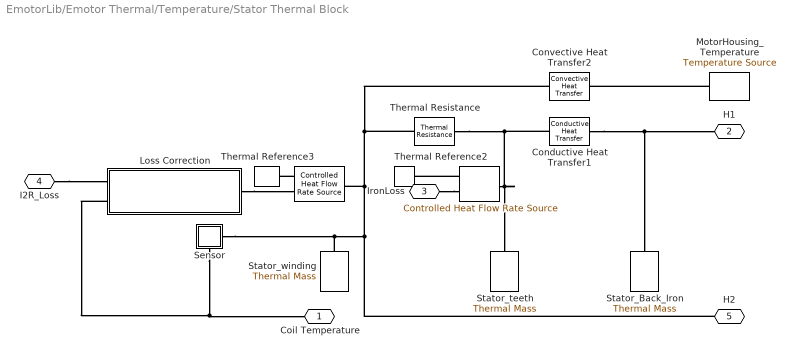
== system EmotorLib/Emotor Thermal/Temperature/Stator Thermal Block ==
  " " : fl_lib/Thermal/Thermal Sources/Controlled Heat Flow Rate Source
  "  " : fl_lib/Thermal/Thermal Sources/Controlled Heat Flow Rate Source
  Conductive Heat Transfer1 : fl_lib/Thermal/Thermal Elements/Conductive Heat Transfer  thermal_type=foundation.enum.ConstantVariableTabulated.Constant  wall_geometry=foundation.enum.ConductionWallGeometry.Cylindrical  area=1e-4 m^2  thickness=0.1 m  d_in=StatorRootDia m  d_out=stator_od m  L=rotorStackLength m  th_cond_min=10 W/(K*m)  th_cond=50 W/(K*m)  th_cond_TLU=[413, 401, 392, 383, 371, 357, 342] W/(K*m)  temp_TLU=[200, 273, 400, 600, 800, 1000, 1200] K  T_specify=off  T_priority=None  T=0 K  T_nominal_specify=off  T_nominal_value=1  T_nominal_unit=K  Q_specify=off  Q_priority=None  Q=0 W  Q_nominal_specify=off  Q_nominal_value=1  Q_nominal_unit=W
  Convective Heat Transfer2 : fl_lib/Thermal/Thermal Elements/Convective Heat Transfer  thermal_type=foundation.enum.constant_variable.constant  area=StatorWindingOhArea m^2  heat_tr_coeff=1 W/(K*m^2)  min_heat_tr_coeff=1e-3 W/(K*m^2)  T_specify=off  T_priority=None  T=0 K  T_nominal_specify=off  T_nominal_value=1  T_nominal_unit=K  Q_specify=off  Q_priority=None  Q=0 W  Q_nominal_specify=off  Q_nominal_value=1  Q_nominal_unit=W
  Loss Correction : Subsystem
  MotorHousing_Temperature : fl_lib/Thermal/Thermal Sources/Temperature Source  temperature=90 degC
  Sensor : Subsystem
      settings: PortSchema="{\"entries\":[{\"content\":{\"sides\":[{\"content\":{\"connectorIds\":[\"LConn1\"]},\"type\":\"ConnectorPlacement.EquallySpacedRectSide\",\"uuid\":\"2a9c4c46-5e98-4ad3-ac1b-1643fab919e9\"},{\"content\":{\"connectorIds\":[],\"side\":\"RIGHT\"},\"type\":\"ConnectorPlacement.EquallySpacedRectSide\",\"uuid\":\"818e06c0-624d-478e-bbcc-fcb04ee6018d\"},{\"content\":{\"connectorIds\":[],\"side\":\"TOP\"},\"type\":\"ConnectorPlacement.EquallySpacedRectSide\",\"uuid\":\"5528f141-53ee-42de-bb84-2bf943b57dce\"},{\"content\":{\"connectorIds\":[\"RConn1\"],\"side\":\"BOTTOM\"},\"type\":\"ConnectorPlacement.EquallySpacedRectSide\",\"uuid\":\"84eb734e-86a3-4614-b5bf-5af47052b8ad\"}]},\"type\":\"ConnectorPlacement.EquallySpacedConnector\",\"uuid\":\"b22b55cd-2470-4ac9-8f94-59072ebe807a\"}],\"packageUris\":[\"http://schema.mathworks.com/mf0/Connector/R2020b\"],\"version\":\"1.0\"}"
  Stator_Back_Iron : fl_lib/Thermal/Thermal Elements/Thermal Mass  mass_type=foundation.enum.constant_variable.constant  mass=StatorBackIronMass kg  sp_heat=IronSpHeat J/(K*kg)  mass_min=1e-6 kg  num_ports=foundation.enum.numPorts2.one  m_specify=off  m_priority=High  m=1 kg  m_nominal_specify=off  m_nominal_value=1  m_nominal_unit=kg  T_specify=on  T_priority=High  T=InitTemp K  T_nominal_specify=off  T_nominal_value=1  T_nominal_unit=K  Q_specify=off  Q_priority=None  Q=0 W  Q_nominal_specify=off  Q_nominal_value=1  Q_nominal_unit=W
  Stator_teeth : fl_lib/Thermal/Thermal Elements/Thermal Mass  mass_type=foundation.enum.constant_variable.constant  mass=GrossToothMass kg  sp_heat=IronSpHeat J/(K*kg)  mass_min=1e-6 kg  num_ports=foundation.enum.numPorts2.one  m_specify=off  m_priority=High  m=1 kg  m_nominal_specify=off  m_nominal_value=1  m_nominal_unit=kg  T_specify=on  T_priority=High  T=InitTemp K  T_nominal_specify=off  T_nominal_value=1  T_nominal_unit=K  Q_specify=off  Q_priority=None  Q=0 W  Q_nominal_specify=off  Q_nominal_value=1  Q_nominal_unit=W
  Stator_winding : fl_lib/Thermal/Thermal Elements/Thermal Mass  mass_type=foundation.enum.constant_variable.constant  mass=WindingMass kg  sp_heat=CopperSpHeat J/(K*kg)  mass_min=1e-6 kg  num_ports=foundation.enum.numPorts2.one  m_specify=off  m_priority=High  m=1 kg  m_nominal_specify=off  m_nominal_value=1  m_nominal_unit=kg  T_specify=on  T_priority=High  T=InitTemp K  T_nominal_specify=off  T_nominal_value=1  T_nominal_unit=K  Q_specify=off  Q_priority=None  Q=0 W  Q_nominal_specify=off  Q_nominal_value=1  Q_nominal_unit=W
  Thermal Reference2 : fl_lib/Thermal/Thermal Elements/Thermal Reference
  Thermal Reference3 : fl_lib/Thermal/Thermal Elements/Thermal Reference
  Thermal Resistance : fl_lib/Thermal/Thermal Elements/Thermal Resistance  resistance=0.1 K/W  T_specify=off  T_priority=None  T=0 K  T_nominal_specify=off  T_nominal_value=1  T_nominal_unit=K  Q_specify=off  Q_priority=None  Q=0 W  Q_nominal_specify=off  Q_nominal_value=1  Q_nominal_unit=W
  Coil Temperature : PMIOPort  Side=Left
  H1 : PMIOPort  Port=2  Side=Left
  IronLoss : PMIOPort  Port=3  Side=Right
  I2R_Loss : PMIOPort  Port=4  Side=Right
  H2 : PMIOPort  Port=5  Side=Left
  connections:
  Conductive Heat Transfer1/RConn1 -- H1/RConn1 -- Stator_Back_Iron/LConn1
  " "/LConn1 -- Conductive Heat Transfer1/LConn1 -- Thermal Resistance/LConn1 -- Stator_teeth/LConn1
  Stator_winding/LConn1 -- H2/RConn1 -- Convective Heat Transfer2/LConn1 -- Thermal Resistance/RConn1 -- "  "/LConn1 -- Sensor/RConn1
  MotorHousing_Temperature/LConn1 -- Convective Heat Transfer2/RConn1
  "  "/RConn2 -- Thermal Reference3/LConn1
  " "/RConn2 -- Thermal Reference2/LConn1
  IronLoss/RConn1 -- " "/RConn1
  Loss Correction/RConn1 -- "  "/RConn1
  Sensor/LConn1 -- Loss Correction/LConn2 -- Coil Temperature/RConn1
  I2R_Loss/RConn1 -- Loss Correction/LConn1

== system EmotorLib/Emotor Thermal/Temperature/Rotor Thermal Block/Sensor ==
  Temperature Sensor : fl_lib/Thermal/Thermal Sensors/Temperature Sensor  temperature_measure=foundation.enum.MeasurementReference.difference
  Thermal Reference1 : fl_lib/Thermal/Thermal Elements/Thermal Reference
  " " : PMIOPort  Side=Left
  "  " : PMIOPort  Port=2  Side=Right
  connections:
  "  "/RConn1 -- Temperature Sensor/RConn2
  Thermal Reference1/LConn1 -- Temperature Sensor/RConn1
  Temperature Sensor/LConn1 -- " "/RConn1

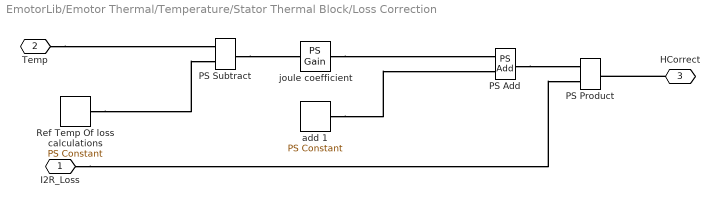
== system EmotorLib/Emotor Thermal/Temperature/Stator Thermal Block/Loss Correction ==
  PS Add : fl_lib/Physical Signals/Functions/PS Add
  PS Product : fl_lib/Physical Signals/Functions/PS Product
  PS Subtract : fl_lib/Physical Signals/Functions/PS Subtract
  Ref Temp Of loss calculations : fl_lib/Physical Signals/Sources/PS Constant  constant=298 K
  add 1 : fl_lib/Physical Signals/Sources/PS Constant  constant=1
  joule coefficient : fl_lib/Physical Signals/Functions/PS Gain  gain=0.00386 1/K
  I2R_Loss : PMIOPort  Side=Left
  Temp : PMIOPort  Port=2  Side=Left
  HCorrect : PMIOPort  Port=3  Side=Right
  connections:
  add 1/RConn1 -- PS Add/LConn2
  Ref Temp Of loss calculations/RConn1 -- PS Subtract/LConn2
  Temp/RConn1 -- PS Subtract/LConn1
  I2R_Loss/RConn1 -- PS Product/LConn2
  PS Add/RConn1 -- PS Product/LConn1
  joule coefficient/RConn1 -- PS Add/LConn1
  PS Subtract/RConn1 -- joule coefficient/LConn1
  HCorrect/RConn1 -- PS Product/RConn1

== system EmotorLib/Emotor Thermal/Temperature/Stator Thermal Block/Sensor ==
  Temperature Sensor : fl_lib/Thermal/Thermal Sensors/Temperature Sensor  temperature_measure=foundation.enum.MeasurementReference.difference
  Thermal Reference1 : fl_lib/Thermal/Thermal Elements/Thermal Reference
  "  " : PMIOPort  Side=Left
  " " : PMIOPort  Port=2  Side=Right
  connections:
  Thermal Reference1/LConn1 -- Temperature Sensor/RConn1
  Temperature Sensor/RConn2 -- "  "/RConn1
  " "/RConn1 -- Temperature Sensor/LConn1
